simulink model "fwc_reference_wrapper"  (R2026a)
settings: Solver=FixedStepDiscrete  FixedStep=5e-4
settings Model: Creator=ASUS  LastModifiedBy=ASUS
settings HardwareCC: ProdLargestAtomicInteger=Long  ProdLargestAtomicFloat=Double  ProdHWDeviceType=ARM Compatible->ARM Cortex-M
settings RTWCC: SystemTargetFile=ert.tlc  GenCodeOnly=on  Description=Embedded Coder
settings ERTTargetCC: GenerateSampleERTMain=on

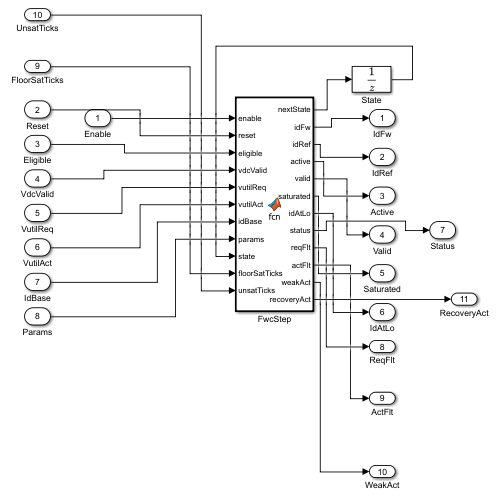
[thumbnail: Simulink's stored preview of the top-level diagram]
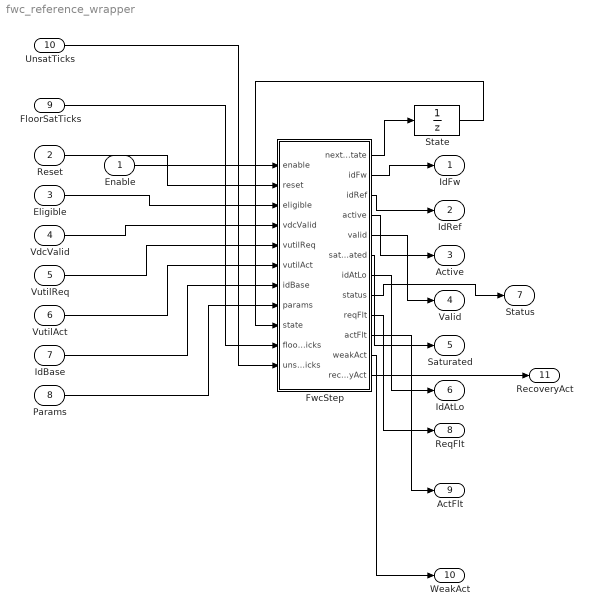
== system fwc_reference_wrapper ==
  Enable : Inport  OutDataTypeStr=uint8
  Reset : Inport  Port=2  OutDataTypeStr=uint8
  Eligible : Inport  Port=3  OutDataTypeStr=uint8
  VdcValid : Inport  Port=4  OutDataTypeStr=uint8
  VutilReq : Inport  Port=5  OutDataTypeStr=single
  VutilAct : Inport  Port=6  OutDataTypeStr=single
  IdBase : Inport  Port=7  OutDataTypeStr=single
  Params : Inport  Port=8  OutDataTypeStr=single  PortDimensions=11
  FloorSatTicks : Inport  Port=9  OutDataTypeStr=uint32  PortDimensions=1
  UnsatTicks : Inport  Port=10  OutDataTypeStr=uint32  PortDimensions=1
  FwcStep : MATLAB Function  TreatAsAtomicUnit=on
  State : UnitDelay  InitialCondition=zeros(16,1,'single')  SampleTime=0.0005
  IdFw : Outport
  IdRef : Outport  Port=2
  Active : Outport  Port=3
  Valid : Outport  Port=4
  Saturated : Outport  Port=5
  IdAtLo : Outport  Port=6
  Status : Outport  Port=7
  ReqFlt : Outport  Port=8
  ActFlt : Outport  Port=9
  WeakAct : Outport  Port=10
  RecoveryAct : Outport  Port=11
  wires:
  Reset/1 -> FwcStep/2(reset)
  Eligible/1 -> FwcStep/3(eligible)
  VdcValid/1 -> FwcStep/4(vdcValid)
  VutilReq/1 -> FwcStep/5(vutilReq)
  VutilAct/1 -> FwcStep/6(vutilAct)
  IdBase/1 -> FwcStep/7(idBase)
  Params/1 -> FwcStep/8(params)
  State/1 -> FwcStep/9(state)
  FwcStep/1(nextState) -> State/1
  FwcStep/2(idFw) -> IdFw/1
  FwcStep/3(idRef) -> IdRef/1
  FwcStep/4(active) -> Active/1
  FwcStep/5(valid) -> Valid/1
  FwcStep/6(saturated) -> Saturated/1
  FwcStep/7(idAtLo) -> IdAtLo/1
  FwcStep/12(recoveryAct) -> RecoveryAct/1
  FwcStep/11(weakAct) -> WeakAct/1
  FwcStep/10(actFlt) -> ActFlt/1
  FwcStep/9(reqFlt) -> ReqFlt/1
  UnsatTicks/1 -> FwcStep/11(unsatTicks)
  FloorSatTicks/1 -> FwcStep/10(floorSatTicks)
  FwcStep/8(status) -> Status/1
  Enable/1 -> FwcStep/1(enable)

== matlab function fwc_reference_wrapper/FwcStep ==
  data: enable input uint8; nextState output single size=[16 1]; reset input uint8; eligible input uint8; vdcValid input uint8; vutilReq input single; vutilAct input single; idBase input single; params input single size=[11 1]; state input single size=[16 1]; idFw output single; idRef output single; active output uint8; valid output uint8; saturated output uint8; idAtLo output uint8; status output uint8; floorSatTicks input; unsatTicks input; reqFlt output; actFlt output; weakAct output; recoveryAct output
function [nextState,idFw,idRef,active,valid,saturated,idAtLo,status,reqFlt,actFlt,weakAct,recoveryAct] = fcn(enable,reset,eligible,vdcValid,vutilReq,vutilAct,idBase,params,state,floorSatTicks,unsatTicks)
%#codegen
[nextState,idFw,idRef,active,valid,saturated,idAtLo,status,reqFlt,actFlt,weakAct,recoveryAct] = fwc_reference_step(enable,reset,eligible,vdcValid,vutilReq,vutilAct,idBase,state,params,floorSatTicks,unsatTicks);
end
